simulink model "shock_motion"  (R2018a)
settings: Solver=ode45  StartTime=0.0  StopTime=15  FixedStep=.1  RelTol=1e-3  EnableMultiTasking=on
PreLoadFcn:
  | Cd=1;
  | Cs=2;
  | M=1;
settings Model: Creator=jrivitus  LastModifiedBy=bneiswan
settings DataIOCC: LimitDataPoints=on  SaveFormat=Array
settings OptimizationCC: ExpressionDepthLimit=2147483647  InitFltsAndDblsToZero=on  LifeSpan=inf
settings DebuggingCC: SaveWithParameterizedLinksMsg=none  UnderspecifiedInitializationDetection=Classic  MergeDetectMultiDrivingBlocksExec=none  SignalResolutionControl=TryResolveAllWithWarning  MultiTaskDSMMsg=warning  MultiTaskCondExecSysMsg=none  ParameterPrecisionLossMsg=none  FcnCallInpInsideContextMsg=warning  AllowSymbolicDim=off  StateNameClashWarn=warning  SFUnexpectedBacktrackingDiag=warning  SFNoUnconditionalDefaultTransitionDiag=warning  SFExecutionAtInitializationDiag=none
settings HardwareCC: ProdBitPerPointer=32  ProdBitPerSizeT=32  ProdBitPerPtrDiffT=32  ProdLargestAtomicFloat=None  ProdIntDivRoundTo=Undefined  ProdEndianess=Unspecified  ProdWordSize=32  ProdHWDeviceType=32-bit Generic
settings ModelReferenceCC: PropagateSignalLabelsOutOfModel=off
settings CodeAppCC: StateflowObjectComments=on
settings GRTTargetCC: TargetFcnLib=ansi_tfl_tmw.mat  TargetLangStandard=C89/C90 (ANSI)  GeneratePreprocessorConditionals=Disable all  CombineOutputUpdateFcns=off  GRTInterface=on
settings ConfigComp: CovMetricSettings=dw  CovHtmlReporting=on  CovSaveCumulativeToWorkspaceVar=on  CovSaveSingleToWorkspaceVar=on  CovExternalEMLEnable=off  CovSFcnEnable=off

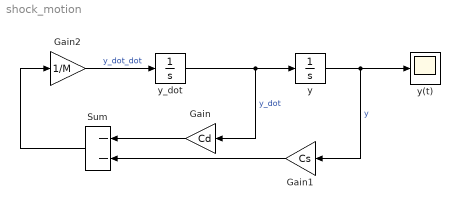
== system shock_motion ==
  Gain : Gain  Gain=Cd
  Gain1 : Gain  Gain=Cs
  Gain2 : Gain  Gain=1/M
  Sum : Sum  Inputs=--
  y : Integrator
      settings: AttributesFormatString=I.C. = %<InitialCondition>
  y(t) : Scope
  y_dot : Integrator  InitialCondition=1
      settings: AttributesFormatString=I.C. = %<InitialCondition>
  wires:
  y/1 -> Gain1/1, y(t)/1  "y"
  y_dot/1 -> y/1, Gain/1  "y_dot"
  Sum/1 -> Gain2/1
  Gain/1 -> Sum/1
  Gain1/1 -> Sum/2
  Gain2/1 -> y_dot/1  "y_dot_dot"
